simulink model "CM620C_MotAg0Meas"  (R2013b)
settings: Solver=FixedStepDiscrete  SolverMode=SingleTasking  StartTime=0.0  StopTime=1  FixedStep=0.0000625  RelTol=1e-3
values from neighbouring files (symbols this model uses):
  ARCHGLBPRM_2PI_ULS_F32 = DataDict.Constant    [CM620C_MotAg0Meas_DataDict.m]
  COEFFTBLELMSIZE_CNT_U08 = DataDict.Constant    [CM620C_MotAg0Meas_DataDict.m]
  COEFFTBLSIZE_CNT_U08 = DataDict.Constant    [CM620C_MotAg0Meas_DataDict.m]
  CORRNTBLAGSTEPSIZE_MATRAD_F32 = DataDict.Constant    [CM620C_MotAg0Meas_DataDict.m]
  CORRNTBLSIDXOFFS_CNT_U16 = DataDict.Constant    [CM620C_MotAg0Meas_DataDict.m]
  CORRNTBLSIZE_CNT_U16 = DataDict.Constant    [CM620C_MotAg0Meas_DataDict.m]
  CORRNTBLSIZEMASK_CNT_U08 = DataDict.Constant    [CM620C_MotAg0Meas_DataDict.m]
  MOTAG0ERRTHD_MOTREV_U0P16 = DataDict.Constant    [CM620C_MotAg0Meas_DataDict.m]
  MotAg0PrtclFlt = DataDict.NTC    [CM620C_MotAg0Meas_DataDict.m]
  MOTAG0PRTCLFLTFAILSTEP_CNT_U16 = DataDict.Constant    [CM620C_MotAg0Meas_DataDict.m]
  MOTAG0PRTCLFLTPASSSTEP_CNT_U16 = DataDict.Constant    [CM620C_MotAg0Meas_DataDict.m]
  MOTAGCPTLIMFLTMASK_CNT_U32 = DataDict.Constant    [CM620C_MotAg0Meas_DataDict.m]
  MOTAGDELTAPERCORRNPT_CNT_U16 = DataDict.Constant    [CM620C_MotAg0Meas_DataDict.m]
  MOTAGFLTMASK_CNT_U32 = DataDict.Constant    [CM620C_MotAg0Meas_DataDict.m]
  MOTAGIDXMASK_CNT_U16 = DataDict.Constant    [CM620C_MotAg0Meas_DataDict.m]
  MOTAGLIMMASK_CNT_S32 = DataDict.Constant    [CM620C_MotAg0Meas_DataDict.m]
  MOTAGMGNLIMFLTMASK_CNT_U32 = DataDict.Constant    [CM620C_MotAg0Meas_DataDict.m]
  MOTAGMINWAITPERD_CNT_U32 = DataDict.Constant    [CM620C_MotAg0Meas_DataDict.m]
  MOTAGOFFS_CNT_S32 = DataDict.Constant    [CM620C_MotAg0Meas_DataDict.m]
  MOTAGOVFFLTMASK_CNT_U32 = DataDict.Constant    [CM620C_MotAg0Meas_DataDict.m]
  MOTAGSPITRSMMASK_CNT_U32 = DataDict.Constant    [CM620C_MotAg0Meas_DataDict.m]
  MOTAGVLTGFLTMASK_CNT_U32 = DataDict.Constant    [CM620C_MotAg0Meas_DataDict.m]
  NOMOTAGFLTMASK_CNT_U32 = DataDict.Constant    [CM620C_MotAg0Meas_DataDict.m]
  READBUFADR_CNT_U32 = DataDict.Constant    [CM620C_MotAg0Meas_DataDict.m]
  READBUFIDX_CNT_U08 = DataDict.Constant    [CM620C_MotAg0Meas_DataDict.m]
  SNSRAGMASK_CNT_U32 = DataDict.Constant    [CM620C_MotAg0Meas_DataDict.m]
  SNSRCNTMASK_CNT_U32 = DataDict.Constant    [CM620C_MotAg0Meas_DataDict.m]
  SPIAGCNTREGIDX_CNT_U08 = DataDict.Constant    [CM620C_MotAg0Meas_DataDict.m]
  SPIAGREGIDX_CNT_U08 = DataDict.Constant    [CM620C_MotAg0Meas_DataDict.m]
  SPISTATREGIDX_CNT_U08 = DataDict.Constant    [CM620C_MotAg0Meas_DataDict.m]
  SPITURNCNTRREGIDX_CNT_U08 = DataDict.Constant    [CM620C_MotAg0Meas_DataDict.m]
  STRTPTRINITVAL_CNT_U32 = DataDict.Constant    [CM620C_MotAg0Meas_DataDict.m]
  STRTPTRPERVAL_CNT_U32 = DataDict.Constant    [CM620C_MotAg0Meas_DataDict.m]
  TURNCNTRHALFOFFS_CNT_S16 = DataDict.Constant    [CM620C_MotAg0Meas_DataDict.m]
  TURNCNTROFFS_CNT_S16 = DataDict.Constant    [CM620C_MotAg0Meas_DataDict.m]
  TURNCNTRREGMASK_CNT_U32 = DataDict.Constant    [CM620C_MotAg0Meas_DataDict.m]
  VLDMOTAGFLTMASK_CNT_U32 = DataDict.Constant    [CM620C_MotAg0Meas_DataDict.m]
undefined symbols (not defined in the file or in its folder): NtcSts1, sigbuilder_block
libraries: simulink x41, FloatToFixd x1, NxtrMax x1
(part 2 of 7)

== system CM620C_MotAg0Meas/MotAg0Meas/MotAg0MeasPer2/MotAg0Calcn ==
  MotAgMecl0Polarity : Inport
  MotAg3Mecl : Inport  Port=2
  MotAg0DiagcAg : Inport  Port=3
  Enable : EnablePort
  CopyRight2 : Subsystem  Description=|  mask(Copyright Information){none=on}
      | Copyright info block.                                               
      |                                                                     
      | Place copyright information at the top of every subsystem in design.
      mask prompts: none "No parameters"
      mask help: Place copyright information at the top of every subsystem in design.
      mask Display:
      | NxtrConf = 'Nexteer Confidential';
      | 
      | sys = bdroot; %handle for the current model ("system")
      | first = get_param(sys,'Created');
      | first = first(end-3:end);  %year is last four digits
      | 
      | last = get_param(sys,'LastModifiedDate');
      | if isempty(last)
      |     last = datestr(now,'yyyy');
      | else
      |     last = last(end-3:end);
      | end
      | 
      | if strcmp(first,last)
      |     fprintf('%s -- Copyright %s Nexteer',NxtrConf,first)
      | else
      |     fprintf('%s -- %s%s- %s Nexteer',NxtrConf,char(169),first,last)
      | end
  MotAg0Processing : Subsystem
  SpiRx : Subsystem  TreatAsAtomicUnit=on
  MotAg0MeclQlfr : Outport  RequirementInfo={} %GIDa_565f93ed_943b_4312_a87f_51762b2a2119
  MotAg0MeclRollgCntr : Outport  RequirementInfo={} %GIDa_8e528acc_6bf2_45f3_8e8a_135e746b0f24  Port=2
  MotAg0Offs : Outport  Port=3
  wires:
  MotAgMecl0Polarity/1 -> MotAg0Processing/2(MotAgMecl0Polarity)
  MotAg3Mecl/1 -> MotAg0Processing/3(MotAg3Mecl)
  MotAg0Processing/1(MotAg0MeclQlfr) -> MotAg0MeclQlfr/1
  MotAg0Processing/2(MotAg0MeclRollgCntr) -> MotAg0MeclRollgCntr/1
  SpiRx/1(MotAg0RawRegBuf) -> MotAg0Processing/1(MotAg0RawRes)
  MotAg0Processing/3(MotAg0Offs) -> MotAg0Offs/1
  MotAg0DiagcAg/1 -> MotAg0Processing/4(MotAg0DiagcAg)

== system CM620C_MotAg0Meas/MotAg0Meas/MotAg0MeasPer3/CopyRight2 ==

== system CM620C_MotAg0Meas/MotAg0Meas/MotAg0MeasPer3/Initial Check ==
  RegInpCSIH1STR0 : Inport
  0:Idle 1:Communicating : simulink/Logic and Bit Operations/Compare To Zero  relop===  OutDataTypeStr=boolean
  128 : Constant  Value=MOTAGSPITRSMMASK_CNT_U32
  CopyRight2 : Subsystem  Description=|  mask(Copyright Information){none=on}
      | Copyright info block.                                               
      |                                                                     
      | Place copyright information at the top of every subsystem in design.
      mask prompts: none "No parameters"
      mask help: Place copyright information at the top of every subsystem in design.
      mask Display:
      | NxtrConf = 'Nexteer Confidential';
      | 
      | sys = bdroot; %handle for the current model ("system")
      | first = get_param(sys,'Created');
      | first = first(end-3:end);  %year is last four digits
      | 
      | last = get_param(sys,'LastModifiedDate');
      | if isempty(last)
      |     last = datestr(now,'yyyy');
      | else
      |     last = last(end-3:end);
      | end
      | 
      | if strcmp(first,last)
      |     fprintf('%s -- Copyright %s Nexteer',NxtrConf,first)
      | else
      |     fprintf('%s -- %s%s- %s Nexteer',NxtrConf,char(169),first,last)
      | end
  Data Store Write : DataStoreWrite  DataStoreName=MotAg0PrevSpiErrFltCntr
  IdleState SendTx : Subsystem  TreatAsAtomicUnit=on
  If : If  IfExpression=u1==1
  InitTxCommunication going on Wait : Subsystem  TreatAsAtomicUnit=on
  Merge : Merge
  Merge1 : Merge
  TSF Bit : simulink/Logic and Bit Operations/Bitwise Operator  logicop=AND  UseBitMask=off  NumInputPorts=2  BitMask=bin2dec('11011001')  BitMaskRealWorld=Stored Integer
  MotAg3Mecl : Outport
  MotAg0DiagcAg : Outport  Port=2
  MotAg0SpiTrsmEna : Outport  Port=3
  wires:
  If/2 -> InitTxCommunication going on Wait/Action
  TSF Bit/1 -> 0:Idle 1:Communicating/1
  128/1 -> TSF Bit/2
  If/1 -> IdleState SendTx/Action
  RegInpCSIH1STR0/1 -> TSF Bit/1
  IdleState SendTx/3(MotAg0SpiTrsmEna) -> Merge/1
  InitTxCommunication going on Wait/1(MotAg0SpiTrsmEna) -> Merge/2
  Merge/1 -> MotAg0SpiTrsmEna/1
  0:Idle 1:Communicating/1 -> If/1
  IdleState SendTx/1(MotAg3Mecl) -> MotAg3Mecl/1
  Merge1/1 -> Data Store Write/1
  IdleState SendTx/4(FltCntr_u16) -> Merge1/1
  InitTxCommunication going on Wait/2(FltCntr_u16) -> Merge1/2
  IdleState SendTx/2(MotAg0DiagcAg) -> MotAg0DiagcAg/1

== system CM620C_MotAg0Meas/Sensor Simulated Values/Signal Processing/Angle Processing ==
  Angle : Inport
  IIFvsSSC Offs : Inport  Port=2
  0-14 bit angle : Product
  Add : Sum  Inputs=+++
  Constant1 : Constant  Value=32767
  Constant5 : Constant  Value=360
  CopyRight2 : Subsystem  Description=|  mask(Copyright Information){none=on}
      | Copyright info block.                                               
      |                                                                     
      | Place copyright information at the top of every subsystem in design.
      mask prompts: none "No parameters"
      mask help: Place copyright information at the top of every subsystem in design.
      mask Display:
      | NxtrConf = 'Nexteer Confidential';
      | 
      | sys = bdroot; %handle for the current model ("system")
      | first = get_param(sys,'Created');
      | first = first(end-3:end);  %year is last four digits
      | 
      | last = get_param(sys,'LastModifiedDate');
      | if isempty(last)
      |     last = datestr(now,'yyyy');
      | else
      |     last = last(end-3:end);
      | end
      | 
      | if strcmp(first,last)
      |     fprintf('%s -- Copyright %s Nexteer',NxtrConf,first)
      | else
      |     fprintf('%s -- %s%s- %s Nexteer',NxtrConf,char(169),first,last)
      | end
  Divide : Product  Inputs=*/
  Fake 15 th Bit : Constant  Value=32768  OutDataTypeStr=double
  Fake Chip Select Bit : Constant  Value=65536  OutDataTypeStr=double
  Math Function : Math  Operator=mod  SaturateOnIntegerOverflow=on
  Sum2 : Sum
  AgReg : Outport
  wires:
  Fake Chip Select Bit/1 -> Add/1
  Fake 15 th Bit/1 -> Add/2
  Add/1 -> AgReg/1
  Constant1/1 -> 0-14 bit angle/2
  Constant5/1 -> Divide/2, Math Function/2
  Math Function/1 -> Divide/1
  Divide/1 -> Sum2/2
  IIFvsSSC Offs/1 -> Sum2/1
  Sum2/1 -> 0-14 bit angle/1
  0-14 bit angle/1 -> Add/3
  Angle/1 -> Math Function/1

== system CM620C_MotAg0Meas/Sensor Simulated Values/Signal Processing/CopyRight2 ==

== system CM620C_MotAg0Meas/Sensor Simulated Values/Signal Processing/SPI Count Angle ==
  Angle : Inport
  IIFvsSSC Offs : Inport  Port=2
  0-13 bit Cnt : Product
  Abs1 : Abs
  Add : Sum  Inputs=+++
  Add1 : Sum
  Constant1 : Constant  Value=16383
  Constant5 : Constant  Value=360
  CopyRight2 : Subsystem  Description=|  mask(Copyright Information){none=on}
      | Copyright info block.                                               
      |                                                                     
      | Place copyright information at the top of every subsystem in design.
      mask prompts: none "No parameters"
      mask help: Place copyright information at the top of every subsystem in design.
      mask Display:
      | NxtrConf = 'Nexteer Confidential';
      | 
      | sys = bdroot; %handle for the current model ("system")
      | first = get_param(sys,'Created');
      | first = first(end-3:end);  %year is last four digits
      | 
      | last = get_param(sys,'LastModifiedDate');
      | if isempty(last)
      |     last = datestr(now,'yyyy');
      | else
      |     last = last(end-3:end);
      | end
      | 
      | if strcmp(first,last)
      |     fprintf('%s -- Copyright %s Nexteer',NxtrConf,first)
      | else
      |     fprintf('%s -- %s%s- %s Nexteer',NxtrConf,char(169),first,last)
      | end
  Divide : Product  Inputs=*/
  Fake 14 th Bit : Constant  Value=16384  OutDataTypeStr=double
  Fake Chip Select Bit : Constant  Value=65536  OutDataTypeStr=double
  Math Function : Math  Operator=mod  SaturateOnIntegerOverflow=on
  Scope{,1..3} (4 alike) : Scope
      Scope settings: YMin=0  YMax=17000  SaveName=ScopeData32
      Scope1 settings: YMin=0  YMax=17000  SaveName=ScopeData17
      Scope2 settings: YMin=0  YMax=17000  SaveName=ScopeData18
      Scope3 settings: YMin=0  YMax=17000  SaveName=ScopeData20
  IIF Cnt : Outport
  wires:
  Angle/1 -> Math Function/1
  Math Function/1 -> Divide/1
  Constant5/1 -> Math Function/2, Divide/2
  Constant1/1 -> 0-13 bit Cnt/2
  Add/1 -> IIF Cnt/1
  Fake 14 th Bit/1 -> Add/2
  Fake Chip Select Bit/1 -> Add/1
  0-13 bit Cnt/1 -> Scope/1, Add/3
  Divide/1 -> Scope1/1, Add1/1
  IIFvsSSC Offs/1 -> Abs1/1
  Add1/1 -> Scope3/1, 0-13 bit Cnt/1, Scope2/1
  Abs1/1 -> Add1/2

== system CM620C_MotAg0Meas/Sensor Simulated Values/Signal Processing/Simulated Enca Angle ==
  Angle : Inport
  IIF vs SSC Flt Actv : Inport  Port=2
  CopyRight2 : Subsystem  Description=|  mask(Copyright Information){none=on}
      | Copyright info block.                                               
      |                                                                     
      | Place copyright information at the top of every subsystem in design.
      mask prompts: none "No parameters"
      mask help: Place copyright information at the top of every subsystem in design.
      mask Display:
      | NxtrConf = 'Nexteer Confidential';
      | 
      | sys = bdroot; %handle for the current model ("system")
      | first = get_param(sys,'Created');
      | first = first(end-3:end);  %year is last four digits
      | 
      | last = get_param(sys,'LastModifiedDate');
      | if isempty(last)
      |     last = datestr(now,'yyyy');
      | else
      |     last = last(end-3:end);
      | end
      | 
      | if strcmp(first,last)
      |     fprintf('%s -- Copyright %s Nexteer',NxtrConf,first)
      | else
      |     fprintf('%s -- %s%s- %s Nexteer',NxtrConf,char(169),first,last)
      | end
  Logical Operator : Logic  Operator=NOT  AllPortsSameDT=off  OutDataTypeStr=boolean
  Scope1 : Scope
      settings: YMin=0  YMax=750  SaveName=ScopeData9
  Subsystem : Subsystem
  IIFAg : Outport
  wires:
  Angle/1 -> Subsystem/1(Angle)
  Subsystem/1(Simulated Angle) -> Scope1/1, IIFAg/1
  IIF vs SSC Flt Actv/1 -> Logical Operator/1
  Logical Operator/1 -> Subsystem/Enable

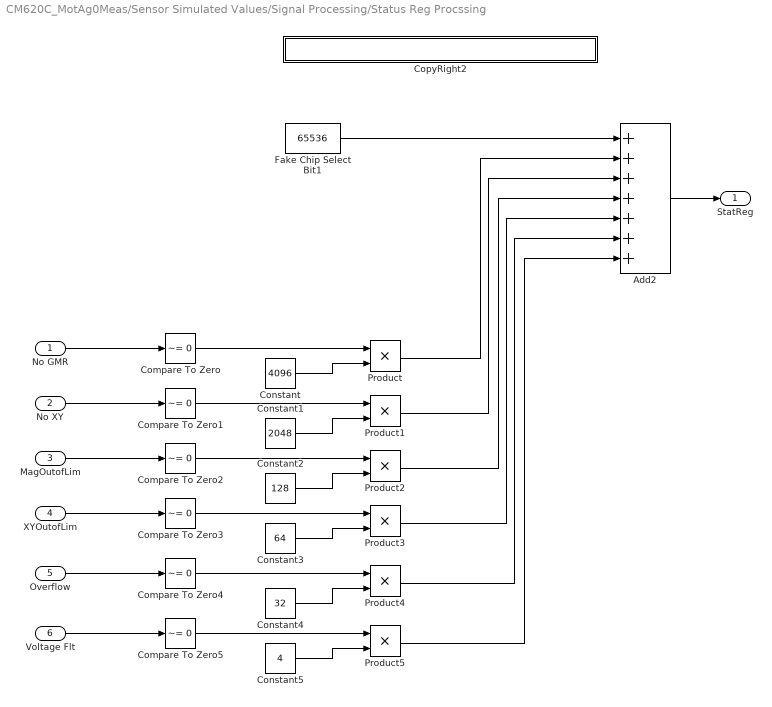
== system CM620C_MotAg0Meas/Sensor Simulated Values/Signal Processing/Status Reg Procssing ==
  No GMR : Inport
  No XY : Inport  Port=2
  MagOutofLim : Inport  Port=3
  XYOutofLim : Inport  Port=4
  Overflow : Inport  Port=5
  Voltage Flt : Inport  Port=6
  Add2 : Sum  Inputs=+++++++
  Compare To Zero{,1..5} (6 alike) : simulink/Logic and Bit Operations/Compare To Zero  relop=~=  OutDataTypeStr=uint8
  Constant : Constant  Value=4096
  Constant1 : Constant  Value=2048
  Constant2 : Constant  Value=128
  Constant3 : Constant  Value=64
  Constant4 : Constant  Value=32
  Constant5 : Constant  Value=4
  CopyRight2 : Subsystem  Description=|  mask(Copyright Information){none=on}
      | Copyright info block.                                               
      |                                                                     
      | Place copyright information at the top of every subsystem in design.
      mask prompts: none "No parameters"
      mask help: Place copyright information at the top of every subsystem in design.
      mask Display:
      | NxtrConf = 'Nexteer Confidential';
      | 
      | sys = bdroot; %handle for the current model ("system")
      | first = get_param(sys,'Created');
      | first = first(end-3:end);  %year is last four digits
      | 
      | last = get_param(sys,'LastModifiedDate');
      | if isempty(last)
      |     last = datestr(now,'yyyy');
      | else
      |     last = last(end-3:end);
      | end
      | 
      | if strcmp(first,last)
      |     fprintf('%s -- Copyright %s Nexteer',NxtrConf,first)
      | else
      |     fprintf('%s -- %s%s- %s Nexteer',NxtrConf,char(169),first,last)
      | end
  Fake Chip Select Bit1 : Constant  Value=65536  OutDataTypeStr=double
  Product{,1..5} (6 alike) : Product
  StatReg : Outport
  wires:
  Fake Chip Select Bit1/1 -> Add2/1
  Add2/1 -> StatReg/1
  Product/1 -> Add2/2
  No GMR/1 -> Compare To Zero/1
  No XY/1 -> Compare To Zero1/1
  MagOutofLim/1 -> Compare To Zero2/1
  XYOutofLim/1 -> Compare To Zero3/1
  Overflow/1 -> Compare To Zero4/1
  Voltage Flt/1 -> Compare To Zero5/1
  Compare To Zero/1 -> Product/1
  Compare To Zero1/1 -> Product1/1
  Compare To Zero2/1 -> Product2/1
  Compare To Zero3/1 -> Product3/1
  Compare To Zero4/1 -> Product4/1
  Compare To Zero5/1 -> Product5/1
  Constant/1 -> Product/2
  Constant1/1 -> Product1/2
  Constant2/1 -> Product2/2
  Constant3/1 -> Product3/2
  Constant4/1 -> Product4/2
  Constant5/1 -> Product5/2
  Product1/1 -> Add2/3
  Product2/1 -> Add2/4
  Product3/1 -> Add2/5
  Product4/1 -> Add2/6
  Product5/1 -> Add2/7

== system CM620C_MotAg0Meas/Sensor Simulated Values/Signal Processing/Turns Counter Processing ==
  Angle : Inport
  Add1 : Sum  Inputs=+++
  Constant1 : Constant  Value=0
  Constant2 : Constant  Value=512
  Constant5 : Constant  Value=360
  CopyRight2 : Subsystem  Description=|  mask(Copyright Information){none=on}
      | Copyright info block.                                               
      |                                                                     
      | Place copyright information at the top of every subsystem in design.
      mask prompts: none "No parameters"
      mask help: Place copyright information at the top of every subsystem in design.
      mask Display:
      | NxtrConf = 'Nexteer Confidential';
      | 
      | sys = bdroot; %handle for the current model ("system")
      | first = get_param(sys,'Created');
      | first = first(end-3:end);  %year is last four digits
      | 
      | last = get_param(sys,'LastModifiedDate');
      | if isempty(last)
      |     last = datestr(now,'yyyy');
      | else
      |     last = last(end-3:end);
      | end
      | 
      | if strcmp(first,last)
      |     fprintf('%s -- Copyright %s Nexteer',NxtrConf,first)
      | else
      |     fprintf('%s -- %s%s- %s Nexteer',NxtrConf,char(169),first,last)
      | end
  Divide1 : Product  Inputs=*/
  Fake 9-15 bits : Constant  Value=65024  OutDataTypeStr=double
  Fake Chip Select Bit : Constant  Value=65536  OutDataTypeStr=double
  Scope : Scope
  Sum1 : Sum
  Switch1 : Switch
  TurnsReg : Outport
  wires:
  Fake 9-15 bits/1 -> Add1/2
  Add1/1 -> TurnsReg/1
  Angle/1 -> Divide1/1
  Fake Chip Select Bit/1 -> Add1/1
  Constant5/1 -> Divide1/2
  Divide1/1 -> Sum1/1, Switch1/2
  Constant1/1 -> Switch1/1
  Constant2/1 -> Switch1/3
  Switch1/1 -> Sum1/2
  Sum1/1 -> Scope/1, Add1/3

== system CM620C_MotAg0Meas/MotAg0Meas/MotAg0MeasInit1/Compute Correction Table/CopyRight2 ==

== system CM620C_MotAg0Meas/MotAg0Meas/MotAg0MeasInit1/Compute Correction Table/MotAg0CoeffTbl_GetErrorStatus ==
  note: 0 simulated for modeling purposes,
      | actual value returned by NVM.  Non-zero return indicates
      | failure in storage/retrievial of NVM.
  Constant : Constant  Value=0
  CopyRight2 : Subsystem  Description=|  mask(Copyright Information){none=on}
      | Copyright info block.                                               
      |                                                                     
      | Place copyright information at the top of every subsystem in design.
      mask prompts: none "No parameters"
      mask help: Place copyright information at the top of every subsystem in design.
      mask Display:
      | NxtrConf = 'Nexteer Confidential';
      | 
      | sys = bdroot; %handle for the current model ("system")
      | first = get_param(sys,'Created');
      | first = first(end-3:end);  %year is last four digits
      | 
      | last = get_param(sys,'LastModifiedDate');
      | if isempty(last)
      |     last = datestr(now,'yyyy');
      | else
      |     last = last(end-3:end);
      | end
      | 
      | if strcmp(first,last)
      |     fprintf('%s -- Copyright %s Nexteer',NxtrConf,first)
      | else
      |     fprintf('%s -- %s%s- %s Nexteer',NxtrConf,char(169),first,last)
      | end
  RequestResultPtr : Outport
  wires:
  Constant/1 -> RequestResultPtr/1

== system CM620C_MotAg0Meas/MotAg0Meas/MotAg0MeasInit1/Compute Correction Table/NVM NOK ==
  note: In the event of a NVM failure
      | set the correction table to 0
  Action Port : ActionPort  ActionType=else
  Constant1 : Constant  Value=CORRNTBLSIZE_CNT_U16
  CopyRight2 : Subsystem  Description=|  mask(Copyright Information){none=on}
      | Copyright info block.                                               
      |                                                                     
      | Place copyright information at the top of every subsystem in design.
      mask prompts: none "No parameters"
      mask help: Place copyright information at the top of every subsystem in design.
      mask Display:
      | NxtrConf = 'Nexteer Confidential';
      | 
      | sys = bdroot; %handle for the current model ("system")
      | first = get_param(sys,'Created');
      | first = first(end-3:end);  %year is last four digits
      | 
      | last = get_param(sys,'LastModifiedDate');
      | if isempty(last)
      |     last = datestr(now,'yyyy');
      | else
      |     last = last(end-3:end);
      | end
      | 
      | if strcmp(first,last)
      |     fprintf('%s -- Copyright %s Nexteer',NxtrConf,first)
      | else
      |     fprintf('%s -- %s%s- %s Nexteer',NxtrConf,char(169),first,last)
      | end
  Zero out correction table : Subsystem  TreatAsAtomicUnit=on
  wires:
  Constant1/1 -> Zero out correction table/1(N)

== system CM620C_MotAg0Meas/MotAg0Meas/MotAg0MeasInit1/Compute Correction Table/NVM Ok ==
  Action Port : ActionPort  ActionType=then
  Calculate Correction Table : Subsystem  Priority=100  TreatAsAtomicUnit=on
      settings: AttributesFormatString=|
      | Priority:
      | %<Priority>
  Configure Coefficients : Subsystem  Priority=10  TreatAsAtomicUnit=on
      settings: AttributesFormatString=|
      | Priority:
      | %<Priority>
  CopyRight2 : Subsystem  Description=|  mask(Copyright Information){none=on}
      | Copyright info block.                                               
      |                                                                     
      | Place copyright information at the top of every subsystem in design.
      mask prompts: none "No parameters"
      mask help: Place copyright information at the top of every subsystem in design.
      mask Display:
      | NxtrConf = 'Nexteer Confidential';
      | 
      | sys = bdroot; %handle for the current model ("system")
      | first = get_param(sys,'Created');
      | first = first(end-3:end);  %year is last four digits
      | 
      | last = get_param(sys,'LastModifiedDate');
      | if isempty(last)
      |     last = datestr(now,'yyyy');
      | else
      |     last = last(end-3:end);
      | end
      | 
      | if strcmp(first,last)
      |     fprintf('%s -- Copyright %s Nexteer',NxtrConf,first)
      | else
      |     fprintf('%s -- %s%s- %s Nexteer',NxtrConf,char(169),first,last)
      | end

== system CM620C_MotAg0Meas/MotAg0Meas/MotAg0MeasInit1/Initialize CSIH Registers and Start Transmission/CopyRight2 ==

== system CM620C_MotAg0Meas/MotAg0Meas/MotAg0MeasPer1/GetRefTmr1MicroSec32bit/CopyRight2 ==

== system CM620C_MotAg0Meas/MotAg0Meas/MotAg0MeasPer1/Motor Angle Processing/CopyRight2 ==

== system CM620C_MotAg0Meas/MotAg0Meas/MotAg0MeasPer1/Motor Angle Processing/GetMotAg3Mecl ==
  CopyRight2 : Subsystem  Description=|  mask(Copyright Information){none=on}
      | Copyright info block.                                               
      |                                                                     
      | Place copyright information at the top of every subsystem in design.
      mask prompts: none "No parameters"
      mask help: Place copyright information at the top of every subsystem in design.
      mask Display:
      | NxtrConf = 'Nexteer Confidential';
      | 
      | sys = bdroot; %handle for the current model ("system")
      | first = get_param(sys,'Created');
      | first = first(end-3:end);  %year is last four digits
      | 
      | last = get_param(sys,'LastModifiedDate');
      | if isempty(last)
      |     last = datestr(now,'yyyy');
      | else
      |     last = last(end-3:end);
      | end
      | 
      | if strcmp(first,last)
      |     fprintf('%s -- Copyright %s Nexteer',NxtrConf,first)
      | else
      |     fprintf('%s -- %s%s- %s Nexteer',NxtrConf,char(169),first,last)
      | end
  Do not code - SimulationOnly : DataStoreRead  DataStoreName=SimulatedIIFAg
  MotAgMecl : Outport
  wires:
  Do not code - SimulationOnly/1 -> MotAgMecl/1

== system CM620C_MotAg0Meas/MotAg0Meas/MotAg0MeasPer1/Motor Angle Processing/Offset  ==
  MotAg3Mecl : Inport
  MotCtrlMotAg0Offs : Inport  RequirementInfo={} %GIDa_bd850cf1_7aad_4f85_9ca0_6a2ea660765b  Port=2
  Add : Sum  Inputs=+-
  Chart : Stateflow chart  TreatAsAtomicUnit=on
  Compensate MechMotPos : Subsystem  RequirementInfo="{'linktype_rmi_doors' '00011b4e (/ESG Group/FDD Module Requirements/EA4 Specific/CM620C_MotAg0Meas)' '#CM620C_78' 'true' 'REQ:  CM620C_78' '' } %GIDa_7e1af811_171e_4f01_9746_2e074d70b9e9"
  CopyRight2 : Subsystem  Description=|  mask(Copyright Information){none=on}
      | Copyright info block.                                               
      |                                                                     
      | Place copyright information at the top of every subsystem in design.
      mask prompts: none "No parameters"
      mask help: Place copyright information at the top of every subsystem in design.
      mask Display:
      | NxtrConf = 'Nexteer Confidential';
      | 
      | sys = bdroot; %handle for the current model ("system")
      | first = get_param(sys,'Created');
      | first = first(end-3:end);  %year is last four digits
      | 
      | last = get_param(sys,'LastModifiedDate');
      | if isempty(last)
      |     last = datestr(now,'yyyy');
      | else
      |     last = last(end-3:end);
      | end
      | 
      | if strcmp(first,last)
      |     fprintf('%s -- Copyright %s Nexteer',NxtrConf,first)
      | else
      |     fprintf('%s -- %s%s- %s Nexteer',NxtrConf,char(169),first,last)
      | end
  Data Type Conversion2 : DataTypeConversion  OutDataTypeStr=int32
  MotCtrlMotAg0Mecl : Outport
  wires:
  Compensate MechMotPos/1(MotCtrlMotAg0Mecl) -> MotCtrlMotAg0Mecl/1
  Data Type Conversion2/1 -> Add/1
  Chart/1(MechMtrPos1_Out) -> Compensate MechMotPos/1(MotAg0OffsCorrd)
  MotAg3Mecl/1 -> Data Type Conversion2/1
  Add/1 -> Chart/1(MechMtrPos1_In)
  MotCtrlMotAg0Offs/1 -> Add/2

== system CM620C_MotAg0Meas/MotAg0Meas/MotAg0MeasPer2/MotAg0Calcn/CopyRight2 ==

== system CM620C_MotAg0Meas/MotAg0Meas/MotAg0MeasPer2/MotAg0Calcn/MotAg0Processing ==
  note: 0 = ReadSTAT
      | 1 = CSQDeselect
      | 2 = WriteCmd12
      | 3 = ReadAVAL
      | 4 = CSQDeselect
      | 5 = WriteCmd13
      | 6 = ReadAREV
      | 7 = CSQDeselect
      | 8 = WriteCmd14
      | 9 = ReadIIFCNT
  MotAg0RawRes : Inport
  MotAgMecl0Polarity : Inport  Port=2
  MotAg3Mecl : Inport  RequirementInfo={} %GIDa_3acf1ec1_a575_44ff_bf35_8424bec73f1e  Port=3
  MotAg0DiagcAg : Inport  Port=4
  CopyRight2 : Subsystem  Description=|  mask(Copyright Information){none=on}
      | Copyright info block.                                               
      |                                                                     
      | Place copyright information at the top of every subsystem in design.
      mask prompts: none "No parameters"
      mask help: Place copyright information at the top of every subsystem in design.
      mask Display:
      | NxtrConf = 'Nexteer Confidential';
      | 
      | sys = bdroot; %handle for the current model ("system")
      | first = get_param(sys,'Created');
      | first = first(end-3:end);  %year is last four digits
      | 
      | last = get_param(sys,'LastModifiedDate');
      | if isempty(last)
      |     last = datestr(now,'yyyy');
      | else
      |     last = last(end-3:end);
      | end
      | 
      | if strcmp(first,last)
      |     fprintf('%s -- Copyright %s Nexteer',NxtrConf,first)
      | else
      |     fprintf('%s -- %s%s- %s Nexteer',NxtrConf,char(169),first,last)
      | end
  Diagnostics : Subsystem  RequirementInfo="{'linktype_rmi_doors' '00011b4e (/ESG Group/FDD Module Requirements/EA4 Specific/CM620C_MotAg0Meas)' '#CM620C_24' 'true' 'REQ:  CM620C_24' '' } %GIDa_fee35126_b80b_44d5_b25d_08a44f8d19b4"
  "Offset Compensation " : Subsystem
  SPI  Motor Angle Calcn : Subsystem  RequirementInfo="{'linktype_rmi_doors' '00011b4e (/ESG Group/FDD Module Requirements/EA4 Specific/CM620C_MotAg0Meas)' '#CM620C_107' 'true' 'REQ:  CM620C_107' '' } %GIDa_e4cea6ea_dced_4bff_ad4d_1a375bb34ccb"
  SPI IIF Motor Angle : Subsystem
  Turns Counter Calcn : Subsystem
  MotAg0MeclQlfr : Outport  RequirementInfo={} %GIDa_54a3f071_f44b_4fac_a51b_467c5cfc91e8
  MotAg0MeclRollgCntr : Outport  RequirementInfo={} %GIDa_274fe542_370f_4f63_85a7_948c83b87af9  Port=2
  MotAg0Offs : Outport  Port=3
  wires:
  MotAg0RawRes/1 -> SPI IIF Motor Angle/1(MotAg0RawRes), Turns Counter Calcn/3(MotAg0TurnCntrReg), Diagnostics/1(MotAg0RawRes), SPI  Motor Angle Calcn/1(MotAg0RawReg)
  MotAgMecl0Polarity/1 -> Turns Counter Calcn/2(MotAgMecl0Polarity), SPI  Motor Angle Calcn/2(MotAgMecl0Polarity)
  Diagnostics/1(MotAg0MeclQlfr) -> MotAg0MeclQlfr/1
  Diagnostics/2(MotAg0MeclRollgCntr) -> MotAg0MeclRollgCntr/1
  SPI  Motor Angle Calcn/1(MotAg0SpiMecl) -> Turns Counter Calcn/1(MotAg0SpiMeclAg), Diagnostics/3(MotAg0SpiMecl), "Offset Compensation "/2(MotAg0SpiMecl)
  MotAg3Mecl/1 -> "Offset Compensation "/1(MotAg3Mecl)
  "Offset Compensation "/1(MotAg0Offs) -> MotAg0Offs/1
  MotAg0DiagcAg/1 -> Diagnostics/2(MotAg0DiagcAg)

== system CM620C_MotAg0Meas/MotAg0Meas/MotAg0MeasPer2/MotAg0Calcn/SpiRx ==
  note: 0 = ReadSTAT
      | 1 = CSQDeselect
      | 2 = WriteCmd12
      | 3 = ReadAVAL
      | 4 = CSQDeselect
      | 5 = WriteCmd13
      | 6 = ReadAREV
      | 7 = CSQDeselect
      | 8 = WriteCmd14
      | 9 = ReadIIFCNT
  note: CSIH1MRWP0
      | Bit 22:16 (7bit value)
      | 001001 = 9
      | Address of the ReadBuffer.
  " Index" : Constant  Value=READBUFIDX_CNT_U08
  Address of Rx 589824 : Constant  Value=READBUFADR_CNT_U32
  CopyRight2 : Subsystem  Description=|  mask(Copyright Information){none=on}
      | Copyright info block.                                               
      |                                                                     
      | Place copyright information at the top of every subsystem in design.
      mask prompts: none "No parameters"
      mask help: Place copyright information at the top of every subsystem in design.
      mask Display:
      | NxtrConf = 'Nexteer Confidential';
      | 
      | sys = bdroot; %handle for the current model ("system")
      | first = get_param(sys,'Created');
      | first = first(end-3:end);  %year is last four digits
      | 
      | last = get_param(sys,'LastModifiedDate');
      | if isempty(last)
      |     last = datestr(now,'yyyy');
      | else
      |     last = last(end-3:end);
      | end
      | 
      | if strcmp(first,last)
      |     fprintf('%s -- Copyright %s Nexteer',NxtrConf,first)
      | else
      |     fprintf('%s -- %s%s- %s Nexteer',NxtrConf,char(169),first,last)
      | end
  Data : Subsystem
  RegOutpCSIH1MRWP0 : Terminator
  MotAg0RawRegBuf : Outport
  wires:
  Address of Rx 589824/1 -> RegOutpCSIH1MRWP0/1
  " Index"/1 -> Data/1(N)
  Data/1(MotAg0RawRegBuf) -> MotAg0RawRegBuf/1

== system CM620C_MotAg0Meas/MotAg0Meas/MotAg0MeasPer3/Initial Check/CopyRight2 ==

== system CM620C_MotAg0Meas/MotAg0Meas/MotAg0MeasPer3/Initial Check/IdleState SendTx ==
  Action Port : ActionPort  ActionType=then
  Constant : Constant  OutDataTypeStr=boolean
  CopyRight2 : Subsystem  Description=|  mask(Copyright Information){none=on}
      | Copyright info block.                                               
      |                                                                     
      | Place copyright information at the top of every subsystem in design.
      mask prompts: none "No parameters"
      mask help: Place copyright information at the top of every subsystem in design.
      mask Display:
      | NxtrConf = 'Nexteer Confidential';
      | 
      | sys = bdroot; %handle for the current model ("system")
      | first = get_param(sys,'Created');
      | first = first(end-3:end);  %year is last four digits
      | 
      | last = get_param(sys,'LastModifiedDate');
      | if isempty(last)
      |     last = datestr(now,'yyyy');
      | else
      |     last = last(end-3:end);
      | end
      | 
      | if strcmp(first,last)
      |     fprintf('%s -- Copyright %s Nexteer',NxtrConf,first)
      | else
      |     fprintf('%s -- %s%s- %s Nexteer',NxtrConf,char(169),first,last)
      | end
  Flt Cntr Ena : Subsystem  TreatAsAtomicUnit=on
  MotAg0Sync : Subsystem
  MotAg3Mecl : Outport
  MotAg0DiagcAg : Outport  Port=2
  MotAg0SpiTrsmEna : Outport  Port=3
  FltCntr_u16 : Outport  Port=4
  wires:
  MotAg0Sync/1(MotAg3Mecl) -> MotAg3Mecl/1
  Constant/1 -> MotAg0SpiTrsmEna/1
  Flt Cntr Ena/1(FltCntr_u16) -> FltCntr_u16/1
  MotAg0Sync/2(MotAg0DiagcAg) -> MotAg0DiagcAg/1

== system CM620C_MotAg0Meas/MotAg0Meas/MotAg0MeasPer3/Initial Check/InitTxCommunication going on Wait ==
  Action Port : ActionPort  ActionType=else
  Constant : Constant  Value=0  OutDataTypeStr=boolean
  CopyRight2 : Subsystem  Description=|  mask(Copyright Information){none=on}
      | Copyright info block.                                               
      |                                                                     
      | Place copyright information at the top of every subsystem in design.
      mask prompts: none "No parameters"
      mask help: Place copyright information at the top of every subsystem in design.
      mask Display:
      | NxtrConf = 'Nexteer Confidential';
      | 
      | sys = bdroot; %handle for the current model ("system")
      | first = get_param(sys,'Created');
      | first = first(end-3:end);  %year is last four digits
      | 
      | last = get_param(sys,'LastModifiedDate');
      | if isempty(last)
      |     last = datestr(now,'yyyy');
      | else
      |     last = last(end-3:end);
      | end
      | 
      | if strcmp(first,last)
      |     fprintf('%s -- Copyright %s Nexteer',NxtrConf,first)
      | else
      |     fprintf('%s -- %s%s- %s Nexteer',NxtrConf,char(169),first,last)
      | end
  "Last Flt Cntr " : Subsystem  TreatAsAtomicUnit=on
  MotAg0SpiTrsmEna : Outport
  FltCntr_u16 : Outport  Port=2
  wires:
  Constant/1 -> MotAg0SpiTrsmEna/1
  "Last Flt Cntr "/1(FltCntr_u16) -> FltCntr_u16/1

== system CM620C_MotAg0Meas/Sensor Simulated Values/Signal Processing/Angle Processing/CopyRight2 ==

== system CM620C_MotAg0Meas/Sensor Simulated Values/Signal Processing/SPI Count Angle/CopyRight2 ==

== system CM620C_MotAg0Meas/Sensor Simulated Values/Signal Processing/Simulated Enca Angle/CopyRight2 ==

== system CM620C_MotAg0Meas/Sensor Simulated Values/Signal Processing/Simulated Enca Angle/Subsystem ==
  Angle : Inport
  Enable : EnablePort
  16 bit Angle : Product
  Constant1 : Constant  Value=65535
  Constant5 : Constant  Value=360
  CopyRight2 : Subsystem  Description=|  mask(Copyright Information){none=on}
      | Copyright info block.                                               
      |                                                                     
      | Place copyright information at the top of every subsystem in design.
      mask prompts: none "No parameters"
      mask help: Place copyright information at the top of every subsystem in design.
      mask Display:
      | NxtrConf = 'Nexteer Confidential';
      | 
      | sys = bdroot; %handle for the current model ("system")
      | first = get_param(sys,'Created');
      | first = first(end-3:end);  %year is last four digits
      | 
      | last = get_param(sys,'LastModifiedDate');
      | if isempty(last)
      |     last = datestr(now,'yyyy');
      | else
      |     last = last(end-3:end);
      | end
      | 
      | if strcmp(first,last)
      |     fprintf('%s -- Copyright %s Nexteer',NxtrConf,first)
      | else
      |     fprintf('%s -- %s%s- %s Nexteer',NxtrConf,char(169),first,last)
      | end
  Data Type Conversion : DataTypeConversion  OutDataTypeStr=uint16
  Divide : Product  Inputs=*/
  Math Function : Math  Operator=mod  SaturateOnIntegerOverflow=on
  Scope1 : Scope
      settings: YMin=0  YMax=70000  SaveName=ScopeData3
  Scope3 : Scope
      settings: YMin=0  YMax=70000  SaveName=ScopeData10
  Simulated Angle : Outport
  wires:
  Math Function/1 -> Divide/1
  Constant5/1 -> Divide/2, Math Function/2
  Angle/1 -> Math Function/1
  16 bit Angle/1 -> Data Type Conversion/1, Scope3/1
  Constant1/1 -> 16 bit Angle/2
  Divide/1 -> Scope1/1, 16 bit Angle/1
  Data Type Conversion/1 -> Simulated Angle/1

== system CM620C_MotAg0Meas/Sensor Simulated Values/Signal Processing/Status Reg Procssing/CopyRight2 ==

== system CM620C_MotAg0Meas/Sensor Simulated Values/Signal Processing/Turns Counter Processing/CopyRight2 ==

== system CM620C_MotAg0Meas/MotAg0Meas/MotAg0MeasInit1/Compute Correction Table/MotAg0CoeffTbl_GetErrorStatus/CopyRight2 ==

== system CM620C_MotAg0Meas/MotAg0Meas/MotAg0MeasInit1/Compute Correction Table/NVM NOK/CopyRight2 ==

== system CM620C_MotAg0Meas/MotAg0Meas/MotAg0MeasInit1/Compute Correction Table/NVM NOK/Zero out correction table ==
  N : Inport
  Assignment : Assignment  IndexMode=Zero-based  IndexOptions=Index vector (port)  Indices=1  OutputSizes=1
  CopyRight2 : Subsystem  Description=|  mask(Copyright Information){none=on}
      | Copyright info block.                                               
      |                                                                     
      | Place copyright information at the top of every subsystem in design.
      mask prompts: none "No parameters"
      mask help: Place copyright information at the top of every subsystem in design.
      mask Display:
      | NxtrConf = 'Nexteer Confidential';
      | 
      | sys = bdroot; %handle for the current model ("system")
      | first = get_param(sys,'Created');
      | first = first(end-3:end);  %year is last four digits
      | 
      | last = get_param(sys,'LastModifiedDate');
      | if isempty(last)
      |     last = datestr(now,'yyyy');
      | else
      |     last = last(end-3:end);
      | end
      | 
      | if strcmp(first,last)
      |     fprintf('%s -- Copyright %s Nexteer',NxtrConf,first)
      | else
      |     fprintf('%s -- %s%s- %s Nexteer',NxtrConf,char(169),first,last)
      | end
  Data Store Read : DataStoreRead  DataStoreName=MotAg0CorrnTbl
  Data Store Write : DataStoreWrite  DataStoreName=MotAg0CorrnTbl
  For Iterator : ForIterator  ResetStates=reset  IterationSource=external  IndexMode=Zero-based  IterationVariableDataType=int16
  Zero : Constant  Value=0  OutDataTypeStr=int8
  wires:
  For Iterator/1 -> Assignment/3
  N/1 -> For Iterator/1
  Data Store Read/1 -> Assignment/1
  Assignment/1 -> Data Store Write/1
  Zero/1 -> Assignment/2

== system CM620C_MotAg0Meas/MotAg0Meas/MotAg0MeasInit1/Compute Correction Table/NVM Ok/Calculate Correction Table ==
  Build Wave : Subsystem  RequirementInfo="{'linktype_rmi_doors' '00011b4e (/ESG Group/FDD Module Requirements/EA4 Specific/CM620C_MotAg0Meas)' '#CM620C_105' 'true' 'REQ:  CM620C_105' '' } %GIDa_0cb6570d_3ff4_4bbc_bc64_891a7d35f255"  TreatAsAtomicUnit=on
  Change Correction Coordinate : Subsystem  RequirementInfo="{'linktype_rmi_doors' '00011b4e (/ESG Group/FDD Module Requirements/EA4 Specific/CM620C_MotAg0Meas)' '#CM620C_106' 'true' 'REQ:  CM620C_106' '' } %GIDa_47ba537e_c47a_41c6_b867_a5547d132bcb"  TreatAsAtomicUnit=on
  CopyRight2 : Subsystem  Description=|  mask(Copyright Information){none=on}
      | Copyright info block.                                               
      |                                                                     
      | Place copyright information at the top of every subsystem in design.
      mask prompts: none "No parameters"
      mask help: Place copyright information at the top of every subsystem in design.
      mask Display:
      | NxtrConf = 'Nexteer Confidential';
      | 
      | sys = bdroot; %handle for the current model ("system")
      | first = get_param(sys,'Created');
      | first = first(end-3:end);  %year is last four digits
      | 
      | last = get_param(sys,'LastModifiedDate');
      | if isempty(last)
      |     last = datestr(now,'yyyy');
      | else
      |     last = last(end-3:end);
      | end
      | 
      | if strcmp(first,last)
      |     fprintf('%s -- Copyright %s Nexteer',NxtrConf,first)
      | else
      |     fprintf('%s -- %s%s- %s Nexteer',NxtrConf,char(169),first,last)
      | end

== system CM620C_MotAg0Meas/MotAg0Meas/MotAg0MeasInit1/Compute Correction Table/NVM Ok/Configure Coefficients ==
  note: This block is for simulation purposes only.
      |
      | The data in shadowed RAM is to be populated
      | by NVM handler
  CopyRight2 : Subsystem  Description=|  mask(Copyright Information){none=on}
      | Copyright info block.                                               
      |                                                                     
      | Place copyright information at the top of every subsystem in design.
      mask prompts: none "No parameters"
      mask help: Place copyright information at the top of every subsystem in design.
      mask Display:
      | NxtrConf = 'Nexteer Confidential';
      | 
      | sys = bdroot; %handle for the current model ("system")
      | first = get_param(sys,'Created');
      | first = first(end-3:end);  %year is last four digits
      | 
      | last = get_param(sys,'LastModifiedDate');
      | if isempty(last)
      |     last = datestr(now,'yyyy');
      | else
      |     last = last(end-3:end);
      | end
      | 
      | if strcmp(first,last)
      |     fprintf('%s -- Copyright %s Nexteer',NxtrConf,first)
      | else
      |     fprintf('%s -- %s%s- %s Nexteer',NxtrConf,char(169),first,last)
      | end
  Data Store Write : DataStoreWrite  DataStoreName=MotAg0CoeffTbl
  temporary harmonic coefficient holder : Constant  Value=[0 0 0.0199999995529651642 0 0 0 0 0 0 0 0 0 0 0 0 0 0 0 0 0 0 0 0 0 0 0]  OutDataTypeStr=single
  wires:
  temporary harmonic coefficient holder/1 -> Data Store Write/1

== system CM620C_MotAg0Meas/MotAg0Meas/MotAg0MeasInit1/Compute Correction Table/NVM Ok/CopyRight2 ==

== system CM620C_MotAg0Meas/MotAg0Meas/MotAg0MeasPer1/Motor Angle Processing/GetMotAg3Mecl/CopyRight2 ==

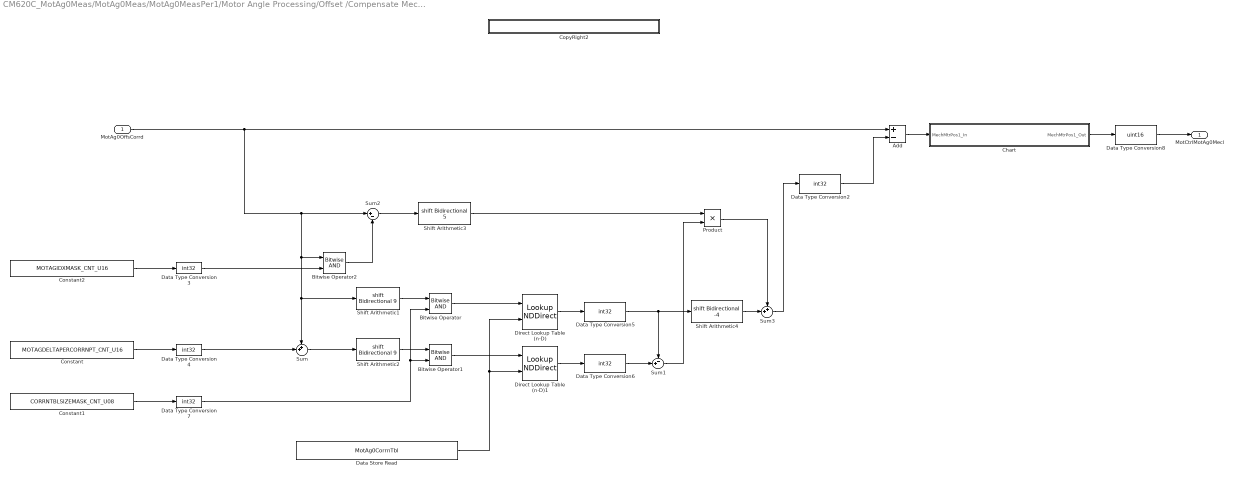
== system CM620C_MotAg0Meas/MotAg0Meas/MotAg0MeasPer1/Motor Angle Processing/Offset /Compensate MechMotPos ==
  MotAg0OffsCorrd : Inport
  Add : Sum  RequirementInfo="{'linktype_rmi_doors' '00011b4e (/ESG Group/FDD Module Requirements/EA4 Specific/CM620C_MotAg0Meas)' '#CM620C_109' 'true' 'REQ:  CM620C_109' '' } %GIDa_19103b05_48c4_4017_a459_e28f509a6931"  Inputs=+-
  Bitwise Operator : simulink/Logic and Bit Operations/Bitwise Operator  logicop=AND  UseBitMask=off  NumInputPorts=2  BitMask=CORRNTBLSIZEMASK_CNT_U08  BitMaskRealWorld=Stored Integer
  Bitwise Operator1 : simulink/Logic and Bit Operations/Bitwise Operator  logicop=AND  UseBitMask=off  NumInputPorts=2  BitMask=CORRNTBLSIZEMASK_CNT_U08  BitMaskRealWorld=Stored Integer
  Bitwise Operator2 : simulink/Logic and Bit Operations/Bitwise Operator  logicop=AND  UseBitMask=off  NumInputPorts=2  BitMask=MOTAGIDXMASK_CNT_U16  BitMaskRealWorld=Stored Integer
  Chart : Stateflow chart  TreatAsAtomicUnit=on
  Constant : Constant  Value=MOTAGDELTAPERCORRNPT_CNT_U16
  Constant1 : Constant  Value=CORRNTBLSIZEMASK_CNT_U08
  Constant2 : Constant  Value=MOTAGIDXMASK_CNT_U16
  CopyRight2 : Subsystem  Description=|  mask(Copyright Information){none=on}
      | Copyright info block.                                               
      |                                                                     
      | Place copyright information at the top of every subsystem in design.
      mask prompts: none "No parameters"
      mask help: Place copyright information at the top of every subsystem in design.
      mask Display:
      | NxtrConf = 'Nexteer Confidential';
      | 
      | sys = bdroot; %handle for the current model ("system")
      | first = get_param(sys,'Created');
      | first = first(end-3:end);  %year is last four digits
      | 
      | last = get_param(sys,'LastModifiedDate');
      | if isempty(last)
      |     last = datestr(now,'yyyy');
      | else
      |     last = last(end-3:end);
      | end
      | 
      | if strcmp(first,last)
      |     fprintf('%s -- Copyright %s Nexteer',NxtrConf,first)
      | else
      |     fprintf('%s -- %s%s- %s Nexteer',NxtrConf,char(169),first,last)
      | end
  Data Store Read : DataStoreRead  DataStoreName=MotAg0CorrnTbl
  Data Type Conversion{2..7} (6 alike) : DataTypeConversion  OutDataTypeStr=int32
  Data Type Conversion8 : DataTypeConversion  OutDataTypeStr=uint16
  Direct Lookup Table (n-D) : LookupNDDirect  NumberOfTableDimensions=1  TableIsInput=on
  Direct Lookup Table (n-D)1 : LookupNDDirect  NumberOfTableDimensions=1  TableIsInput=on
  Product : Product
  Shift Arithmetic1 : ArithShift  BitShiftNumber=9
  Shift Arithmetic2 : ArithShift  BitShiftNumber=9
  Shift Arithmetic3 : ArithShift  BitShiftNumber=5
  Shift Arithmetic4 : ArithShift  BitShiftNumber=-4
  Sum : Sum  Inputs=++|
  Sum1 : Sum  Inputs=-+|
  Sum2 : Sum  Inputs=|+-
  Sum3 : Sum  Inputs=++|
  MotCtrlMotAg0Mecl : Outport
  wires:
  Add/1 -> Chart/1(MechMtrPos1_In)
  Shift Arithmetic1/1 -> Bitwise Operator/1
  Data Type Conversion2/1 -> Add/2
  Chart/1(MechMtrPos1_Out) -> Data Type Conversion8/1
  Sum/1 -> Shift Arithmetic2/1
  Bitwise Operator/1 -> Direct Lookup Table (n-D)/1
  Shift Arithmetic2/1 -> Bitwise Operator1/1
  Bitwise Operator1/1 -> Direct Lookup Table (n-D)1/1
  Data Store Read/1 -> Direct Lookup Table (n-D)/2, Direct Lookup Table (n-D)1/2
  Direct Lookup Table (n-D)/1 -> Data Type Conversion5/1
  Direct Lookup Table (n-D)1/1 -> Data Type Conversion6/1
  Data Type Conversion5/1 -> Shift Arithmetic4/1, Sum1/1
  Data Type Conversion6/1 -> Sum1/2
  Bitwise Operator2/1 -> Sum2/2
  Sum2/1 -> Shift Arithmetic3/1
  Shift Arithmetic3/1 -> Product/1
  Sum1/1 -> Product/2
  Product/1 -> Sum3/1
  Shift Arithmetic4/1 -> Sum3/2
  Sum3/1 -> Data Type Conversion2/1
  Constant1/1 -> Data Type Conversion7/1
  Data Type Conversion7/1 -> Bitwise Operator1/2, Bitwise Operator/2
  Constant2/1 -> Data Type Conversion3/1
  Constant/1 -> Data Type Conversion4/1
  Data Type Conversion3/1 -> Bitwise Operator2/2
  Data Type Conversion4/1 -> Sum/2
  MotAg0OffsCorrd/1 -> Add/1, Sum2/1, Bitwise Operator2/1, Shift Arithmetic1/1, Sum/1
  Data Type Conversion8/1 -> MotCtrlMotAg0Mecl/1

== system CM620C_MotAg0Meas/MotAg0Meas/MotAg0MeasPer1/Motor Angle Processing/Offset /CopyRight2 ==

== system CM620C_MotAg0Meas/MotAg0Meas/MotAg0MeasPer2/MotAg0Calcn/MotAg0Processing/CopyRight2 ==
